simulink model "adative_control_test"  (R2021a)
settings: Solver=VariableStepAuto  StartTime=0.0  StopTime=1000  RelTol=1e-3
settings Model: Creator=pyi12  LastModifiedBy=pyi12

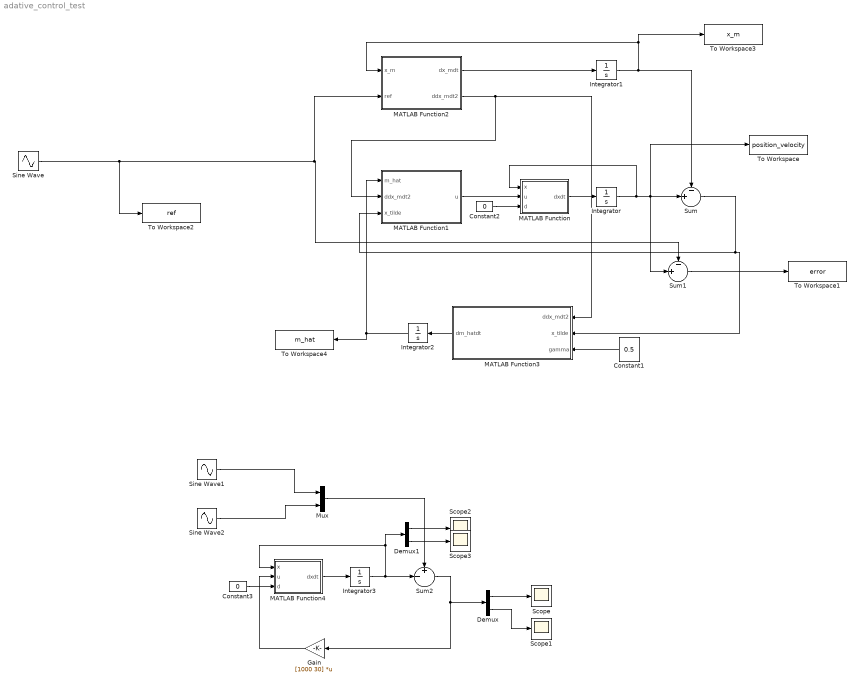
== system adative_control_test ==
  Constant1 : Constant  Value=0.5
  Constant2 : Constant  Value=0
  Constant3 : Constant  Value=0
  Demux : Demux  Outputs=2
  Demux1 : Demux  Outputs=2
  Gain : Gain  Gain=[1000 30]  Multiplication=Matrix(K*u)
  Integrator : Integrator  InitialCondition=[0;0]
  Integrator1 : Integrator  InitialCondition=[0;0]
  Integrator2 : Integrator
  Integrator3 : Integrator  InitialCondition=[0;0]
  MATLAB Function : MATLAB Function  TreatAsAtomicUnit=on
  MATLAB Function1 : MATLAB Function  TreatAsAtomicUnit=on
  MATLAB Function2 : MATLAB Function  TreatAsAtomicUnit=on
  MATLAB Function3 : MATLAB Function  TreatAsAtomicUnit=on
  MATLAB Function4 : MATLAB Function  TreatAsAtomicUnit=on
  Mux : Mux  Inputs=2
  Scope{,1..3} (4 alike) : Scope
  Sine Wave : Sin  Frequency=0.01  SampleTime=0
  Sine Wave1 : Sin  Frequency=4  SampleTime=0
  Sine Wave2 : Sin  Frequency=4  Phase=pi/2  SampleTime=0
  Sum : Sum  Inputs=-|+||
  Sum1 : Sum  Inputs=-|+||
  Sum2 : Sum  Inputs=+|-||
  To Workspace : ToWorkspace  VariableName=position_velocity  SaveFormat=Timeseries  SampleTime=-1
  To Workspace1 : ToWorkspace  VariableName=error  SaveFormat=Timeseries  SampleTime=-1
  To Workspace2 : ToWorkspace  VariableName=ref  SaveFormat=Timeseries  SampleTime=-1
  To Workspace3 : ToWorkspace  VariableName=x_m  SaveFormat=Timeseries  SampleTime=-1
  To Workspace4 : ToWorkspace  VariableName=m_hat  SaveFormat=Timeseries  SampleTime=-1
  wires:
  MATLAB Function/1(dxdt) -> Integrator/1
  Integrator/1 -> To Workspace/1, Sum/2, Sum1/2, MATLAB Function/1(x)
  MATLAB Function1/1(u) -> MATLAB Function/2(u)
  MATLAB Function2/1(dx_mdt) -> Integrator1/1
  Integrator1/1 -> Sum/1, To Workspace3/1, MATLAB Function2/1(x_m)
  MATLAB Function2/2(ddx_mdt2) -> MATLAB Function3/1(ddx_mdt2), MATLAB Function1/2(ddx_mdt2)
  MATLAB Function3/1(dm_hatdt) -> Integrator2/1
  Integrator2/1 -> To Workspace4/1, MATLAB Function1/1(m_hat)
  Sum/1 -> MATLAB Function3/2(x_tilde), MATLAB Function1/3(x_tilde)
  Constant1/1 -> MATLAB Function3/3(gamma)
  Sine Wave/1 -> Sum1/1, MATLAB Function2/2(ref), To Workspace2/1
  Constant2/1 -> MATLAB Function/3(d)
  Sum1/1 -> To Workspace1/1
  MATLAB Function4/1(dxdt) -> Integrator3/1
  Constant3/1 -> MATLAB Function4/3(d)
  Gain/1 -> MATLAB Function4/2(u)
  Sum2/1 -> Demux/1, Gain/1
  Demux/1 -> Scope/1
  Demux/2 -> Scope1/1
  Sine Wave1/1 -> Mux/1
  Mux/1 -> Sum2/1
  Sine Wave2/1 -> Mux/2
  Integrator3/1 -> Sum2/2, MATLAB Function4/1(x), Demux1/1
  Demux1/1 -> Scope2/1
  Demux1/2 -> Scope3/1

== matlab function adative_control_test/MATLAB Function1 ==
  data: m_hat input; ddx_mdt2 input; x_tilde input; u output
function u = controller(m_hat,ddx_mdt2,x_tilde)
lambda = 6;
m_hat = 100;
u = m_hat*(ddx_mdt2 -2*lambda*x_tilde(2) - lambda^2*x_tilde(1));

end

== matlab function adative_control_test/MATLAB Function ==
  data: x input; u input; dxdt output; d input
function dxdt = plant(x,u,d)

m = 100;

A = [0 1;
    0 0];

B = [0;1/m];

dxdt = A*x+B*u+B*d;
end

== matlab function adative_control_test/MATLAB Function2 ==
  data: x_m input; ref input; dx_mdt output; ddx_mdt2 output
function [dx_mdt, ddx_mdt2]= ref_model(x_m,ref)

lambda = [10;25];

A = [0 1;
    -lambda(2) -lambda(1)];
B = [0;lambda(2)];

dx_mdt = A*x_m + B*ref;
ddx_mdt2 = dx_mdt(2);
end

== matlab function adative_control_test/MATLAB Function3 ==
  data: ddx_mdt2 input; x_tilde input; dm_hatdt output; gamma input
function dm_hatdt = adpatation(ddx_mdt2,x_tilde,gamma)

lambda = 6;
s = x_tilde(2) + lambda*x_tilde(1);
v = ddx_mdt2-2*lambda*x_tilde(2) - lambda^2*x_tilde(1);
dm_hatdt = - gamma*v*s;

end

== matlab function adative_control_test/MATLAB Function4 ==
  data: x input; u input; dxdt output; d input
function dxdt = plant(x,u,d)

m = 2;

A = [0 1;
    0 0];

B = [0;1/m];

dxdt = A*x+B*u+B*d;
end
